simulink model "intro_sim_c"  (R2021b)
settings: Solver=VariableStepAuto  StartTime=0.0  StopTime=10.0  RelTol=1e-3
settings Model: Creator=Juho  LastModifiedBy=Juho

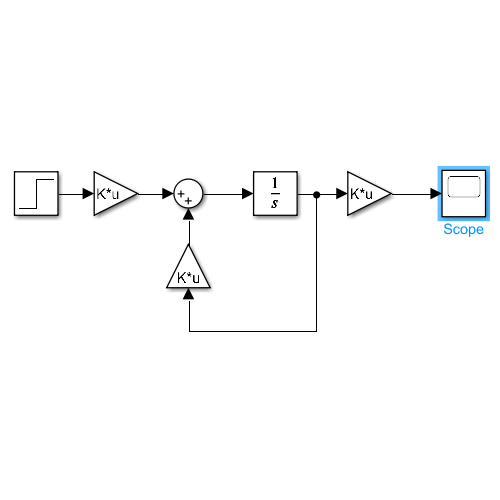
[thumbnail: Simulink's stored preview of the top-level diagram]
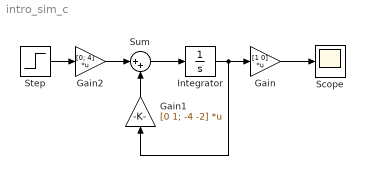
== system intro_sim_c ==
  Gain : Gain  Gain=[1 0]  Multiplication=Matrix(K*u)
  Gain1 : Gain  Gain=[0 1; -4 -2]  Multiplication=Matrix(K*u)
  Gain2 : Gain  Gain=[0; 4]  Multiplication=Matrix(K*u)
  Integrator : Integrator
  Scope : Scope
  Step : Step  Time=0  SampleTime=0
  Sum : Sum  Inputs=|++
  wires:
  Gain/1 -> Scope/1
  Integrator/1 -> Gain1/1, Gain/1
  Sum/1 -> Integrator/1
  Step/1 -> Gain2/1
  Gain1/1 -> Sum/2
  Gain2/1 -> Sum/1
